simulink model "simulation"  (R2023a)
settings: Solver=ode4  StartTime=0.0  StopTime=10.0  FixedStep=.001  RelTol=1e-3
undefined symbols (not defined in the file): k
settings Model: Creator=jackr  LastModifiedBy=jackr

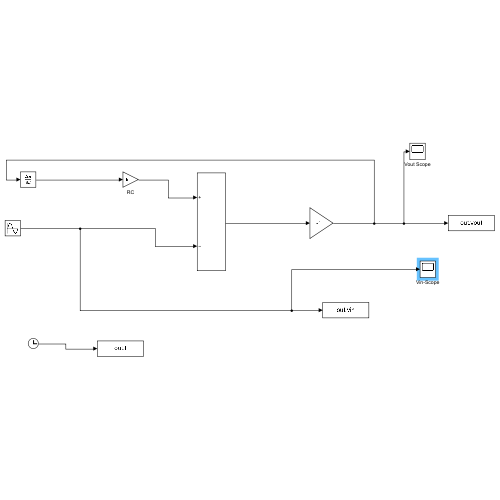
[thumbnail: Simulink's stored preview of the top-level diagram]
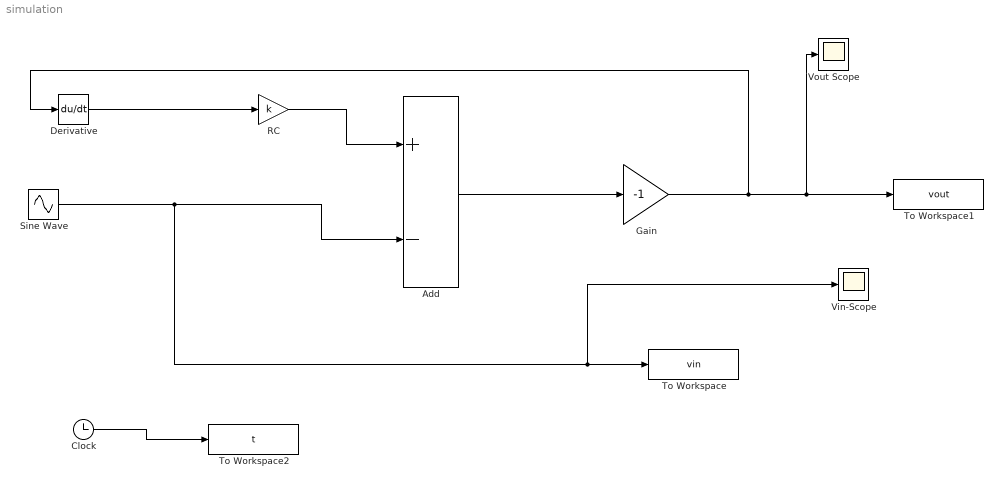
== system simulation ==
  Add : Sum  Inputs=+-
  Clock : Clock
  Derivative : Derivative
  Gain : Gain  Gain=-1
  RC : Gain  Gain=k
  Sine Wave : Sin  Frequency=2*pi * 50  Phase=pi/2  SampleTime=0
  To Workspace : ToWorkspace  VariableName=vin  SaveFormat=Timeseries  SampleTime=-1
  To Workspace1 : ToWorkspace  VariableName=vout  SaveFormat=Timeseries  SampleTime=-1
  To Workspace2 : ToWorkspace  VariableName=t  SaveFormat=Timeseries  SampleTime=-1
  Vin-Scope : Scope
  Vout Scope : Scope
  wires:
  Derivative/1 -> RC/1
  RC/1 -> Add/1
  Add/1 -> Gain/1
  Gain/1 -> Derivative/1, Vout Scope/1, To Workspace1/1
  Clock/1 -> To Workspace2/1
  Sine Wave/1 -> Vin-Scope/1, To Workspace/1, Add/2
